simulink model "amicas_simulator_v1"  (R2024b)
settings: Solver=ode3  StartTime=0.0  StopTime=Tsim  FixedStep=ST  RelTol=1e-3
values from neighbouring files (symbols this model uses):
  alpha_GN = 7.76    [amicas_anesthesia_model.m]
  alpha_RG = 0.33    [amicas_anesthesia_model.m]
  alpha_RGN = 1.61    [amicas_anesthesia_model.m]
  Anest_loop = 1    [amicas_main_program.m]
  Ap = sys11.A    [amicas_estimation_adaptation.m]
  Ar = sys12.A    [amicas_estimation_adaptation.m]
  beta_M = 10.74    [amicas_anesthesia_model.m]
  beta_MN = 3.36    [amicas_anesthesia_model.m]
  Bp = sys11.B    [amicas_estimation_adaptation.m]
  Br = sys12.B    [amicas_estimation_adaptation.m]
  C50N = 3.2425    [amicas_anesthesia_model.m]
  C50P_GN = 1273.3    [amicas_anesthesia_model.m]
  C50P_M = 7.53    [amicas_anesthesia_model.m]
  C50P_MN = 1188.7    [amicas_anesthesia_model.m]
  C50P_RG = 8.26    [amicas_anesthesia_model.m]
  C50P_RGN = 67.77    [amicas_anesthesia_model.m]
  C50Pco = 8    [amicas_hemodyn_model.m]
  C50Pmap = 6    [amicas_hemodyn_model.m]
  C50R_GN = 8.30    (= 8.3)    [amicas_anesthesia_model.m]
  C50R_M = 160.25    [amicas_anesthesia_model.m]
  C50R_MN = 14.64    [amicas_anesthesia_model.m]
  C50Rco = 12    [amicas_hemodyn_model.m]
  C50Rmap = 17    [amicas_hemodyn_model.m]
  Cobasis = 5    [amicas_hemodyn_model.m]
  Cp = sys11.C    [amicas_estimation_adaptation.m]
  Cr = sys12.C    [amicas_estimation_adaptation.m]
  Dist_type = 1    [amicas_main_program.m]
  E0_G = 93.97    [amicas_anesthesia_model.m]
  E0_GN = 33.34    [amicas_anesthesia_model.m]
  E0_M = 93.97    [amicas_anesthesia_model.m]
  E0_MN = 34.48    [amicas_anesthesia_model.m]
  E0_RG = 93.97    [amicas_anesthesia_model.m]
  E0_RGN = 33.69    [amicas_anesthesia_model.m]
  Emax_G = E0_G    (= 93.97)    [amicas_anesthesia_model.m]
  Emax_GN = E0_GN    (= 33.34)    [amicas_anesthesia_model.m]
  Emax_M = E0_M    (= 93.97)    [amicas_anesthesia_model.m]
  Emax_MN = E0_MN    (= 34.48)    [amicas_anesthesia_model.m]
  Emax_RG = E0_RG    (= 93.97)    [amicas_anesthesia_model.m]
  Emax_RGN = E0_RGN    (= 33.69)    [amicas_anesthesia_model.m]
  EmaxPco = 5    [amicas_hemodyn_model.m]
  EmaxPmap = 5    [amicas_hemodyn_model.m]
  EmaxRco = 5    [amicas_hemodyn_model.m]
  EmaxRmap = 15    [amicas_hemodyn_model.m]
  gainPco = 10    [amicas_hemodyn_model.m]
  gainPmap = 15    [amicas_hemodyn_model.m]
  gainRco = 10    [amicas_hemodyn_model.m]
  gainRmap = 10    [amicas_hemodyn_model.m]
  gamma_GN = 7.14    [amicas_anesthesia_model.m]
  gamma_M = 4.13    [amicas_anesthesia_model.m]
  gamma_MN = 6.56    [amicas_anesthesia_model.m]
  gamma_RG = 3.59    [amicas_anesthesia_model.m]
  gamma_RGN = 5.34    [amicas_anesthesia_model.m]
  gammaN = 2.6677    [amicas_anesthesia_model.m]
  gammaPco = 4.5    [amicas_hemodyn_model.m]
  gammaPmap = 4.5    [amicas_hemodyn_model.m]
  gammaRco = 4.5    [amicas_hemodyn_model.m]
  gammaRmap = 4.5    [amicas_hemodyn_model.m]
  k0Pco = 0.81    [amicas_hemodyn_model.m]
  k0Pmap = 0.81    [amicas_hemodyn_model.m]
  k0Rco = 0.51    [amicas_hemodyn_model.m]
  k0Rmap = 0.31    [amicas_hemodyn_model.m]
  k1Pco = 0.81/60    (= 0.0135)    [amicas_hemodyn_model.m]
  k1Pmap = 0.61/60    (= 0.0101666666667)    [amicas_hemodyn_model.m]
  k1Rco = 0.51/60    (= 0.0085)    [amicas_hemodyn_model.m]
  k1Rmap = 0.31/60    (= 0.00516666666667)    [amicas_hemodyn_model.m]
  MAPbasis = 80    [amicas_hemodyn_model.m]
  patient = Patients(index)    [amicas_main_program.m]
  RSM_type = 3    [amicas_main_program.m]
  Ts = 1/60    (= 0.0166666666667)    [amicas_main_program.m]
  Tsc = 5/60    (= 0.0833333333333)    [amicas_estimation_adaptation.m]
libraries: cstblocks x12
settings Model: Creator=Merigo  LastModifiedBy=erhan
settings SolverCC: AlgebraicLoopSolver=TrustRegion
settings DataIOCC: LimitDataPoints=on  SaveFormat=Array  SignalLoggingSaveFormat=ModelDataLogs  ReturnWorkspaceOutputs=off
settings OptimizationCC: BlockReduction=off  BooleanDataType=off  ReuseModelBlockBuffer=off  ExpressionDepthLimit=2147483647  LifeSpan=inf
settings DebuggingCC: SaveWithParameterizedLinksMsg=none  UnderspecifiedInitializationDetection=Classic  MergeDetectMultiDrivingBlocksExec=none  SignalResolutionControl=TryResolveAllWithWarning  MultiTaskDSMMsg=warning  MultiTaskCondExecSysMsg=none  UnconnectedInputMsg=warning  UnconnectedOutputMsg=warning  UnconnectedLineMsg=warning  StateNameClashWarn=warning  SFUnexpectedBacktrackingDiag=warning  SFNoUnconditionalDefaultTransitionDiag=warning  SFExecutionAtInitializationDiag=none  ArithmeticOperatorsInVariantConditions=warning
settings HardwareCC: ProdBitPerPointer=32  ProdBitPerSizeT=32  ProdBitPerPtrDiffT=32  ProdLargestAtomicFloat=None  ProdIntDivRoundTo=Undefined  ProdEndianess=Unspecified  ProdWordSize=32  ProdHWDeviceType=32-bit Generic  TargetUnknown=on
settings ModelReferenceCC: EnableRefExpFcnMdlSchedulingChecks=on  PropagateSignalLabelsOutOfModel=off
settings SFSimCC: SimUseLocalCustomCode=off  CustomCodeUndefinedFunction=UseInterfaceOnly
settings RTWCC: RTWUseLocalCustomCode=off  GPUComputeCapability=3.5  DLArmComputeVersion=19.05
settings CodeAppCC: StateflowObjectComments=on
settings GRTTargetCC: TargetLangStandard=C89/C90 (ANSI)
settings ConfigComp: CovMetricSettings=dw  CovSaveCumulativeToWorkspaceVar=on  CovSaveSingleToWorkspaceVar=on  CovExternalEMLEnable=off

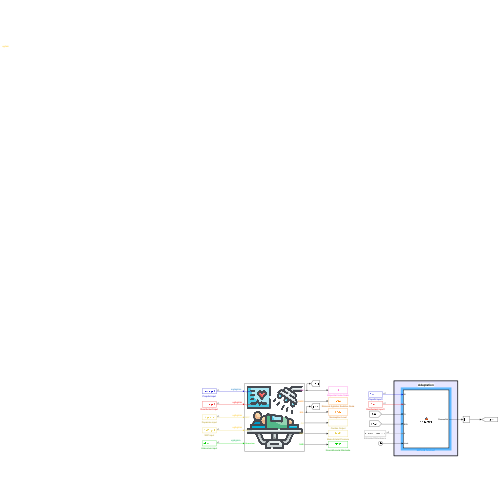
[thumbnail: Simulink's stored preview of the top-level diagram]
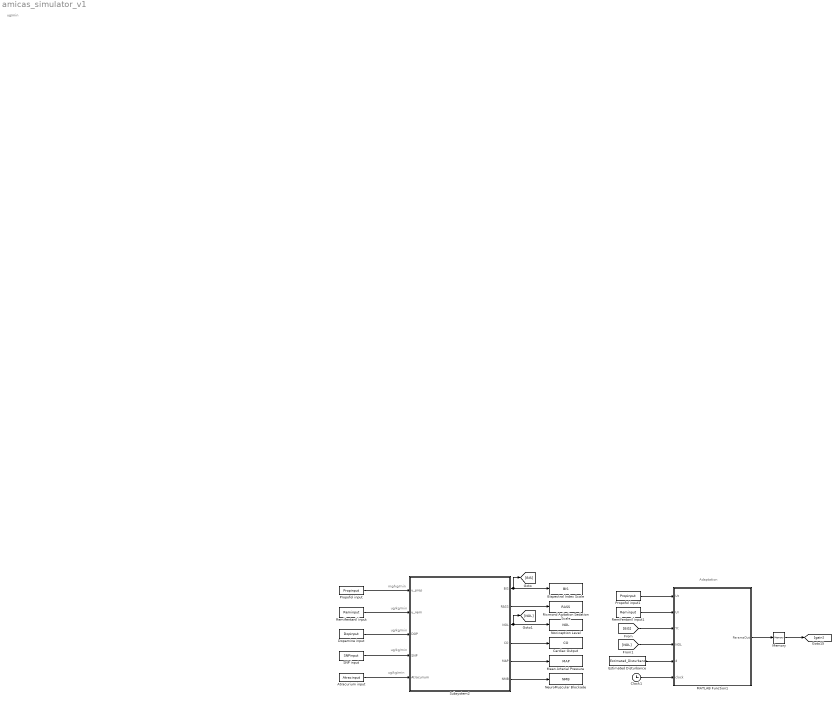
== system amicas_simulator_v1 ==
  note: ug/kg/min
  note: mg/kg/min
  note: ug/min
  note: ug/kg/min
  note: ug/kg/min
  note: ug/kg/min
  note: Adaptation
  Atracurium input : FromWorkspace  VariableName=Atracinput  Interpolate=off  OutputAfterFinalValue=Setting to zero
  Bispectral Index Scale : ToWorkspace  VariableName=BIS  SaveFormat=Timeseries  SampleTime=-1
  Cardiac Output : ToWorkspace  VariableName=CO  SaveFormat=Timeseries  SampleTime=-1
  Clock1 : Clock
  Dopamine input : FromWorkspace  VariableName=Dopinput  Interpolate=off  OutputAfterFinalValue=Setting to zero
  Estimated Disturbance : FromWorkspace  VariableName=Estimated_Disturbance  Interpolate=off  OutputAfterFinalValue=Setting to zero
  MATLAB Function1 : MATLAB Function  TreatAsAtomicUnit=on  SystemSampleTime=Tsc
  Mean Arterial Pressure : ToWorkspace  VariableName=MAP  SaveFormat=Timeseries  SampleTime=-1
  Memory : Memory
  NeuroMuscular Blockade : ToWorkspace  VariableName=NMB  SaveFormat=Timeseries  SampleTime=-1
  Nociception Level : ToWorkspace  VariableName=NOL  SaveFormat=Timeseries  SampleTime=-1
  Propofol input : FromWorkspace  VariableName=Propinput  Interpolate=off  OutputAfterFinalValue=Setting to zero
  Propofol input1 : FromWorkspace  VariableName=Propinput  Interpolate=off  OutputAfterFinalValue=Setting to zero
  Remifentanil input : FromWorkspace  VariableName=Reminput  Interpolate=off  OutputAfterFinalValue=Setting to zero
  Remifentanil input1 : FromWorkspace  VariableName=Reminput  Interpolate=off  OutputAfterFinalValue=Setting to zero
  Ricmond Agitation Sedation Scale : ToWorkspace  VariableName=RASS  SaveFormat=Timeseries  SampleTime=-1
  SNP input : FromWorkspace  VariableName=SNPinput  Interpolate=off  OutputAfterFinalValue=Setting to zero
  Subsystem2 : Subsystem
      mask Display: image('$imagefile');
  wires:
  Propofol input/1 -> Subsystem2/1(u_prop)
  Subsystem2/2(RASS) -> Ricmond Agitation Sedation Scale/1
  Subsystem2/4(CO) -> Cardiac Output/1
  Subsystem2/5(MAP) -> Mean Arterial Pressure/1
  Subsystem2/6(NMB) -> NeuroMuscular Blockade/1
  Atracurium input/1 -> Subsystem2/5(Atracurium)
  Subsystem2/1(BIS) -> Bispectral Index Scale/1, [BIS]
  Remifentanil input/1 -> Subsystem2/2(u_remi)
  Dopamine input/1 -> Subsystem2/3(DOP)
  SNP input/1 -> Subsystem2/4(SNP)
  Subsystem2/3(NOL) -> Nociception Level/1, [NOL]
  [NOL] -> MATLAB Function1/4(NOL)
  [BIS] -> MATLAB Function1/3(Yt)
  Propofol input1/1 -> MATLAB Function1/1(Ut)
  Memory/1 -> [gain]
  MATLAB Function1/1(ParamsOut) -> Memory/1
  Clock1/1 -> MATLAB Function1/6(clock)
  Estimated Disturbance/1 -> MATLAB Function1/5(d)
  Remifentanil input1/1 -> MATLAB Function1/2(Ur)

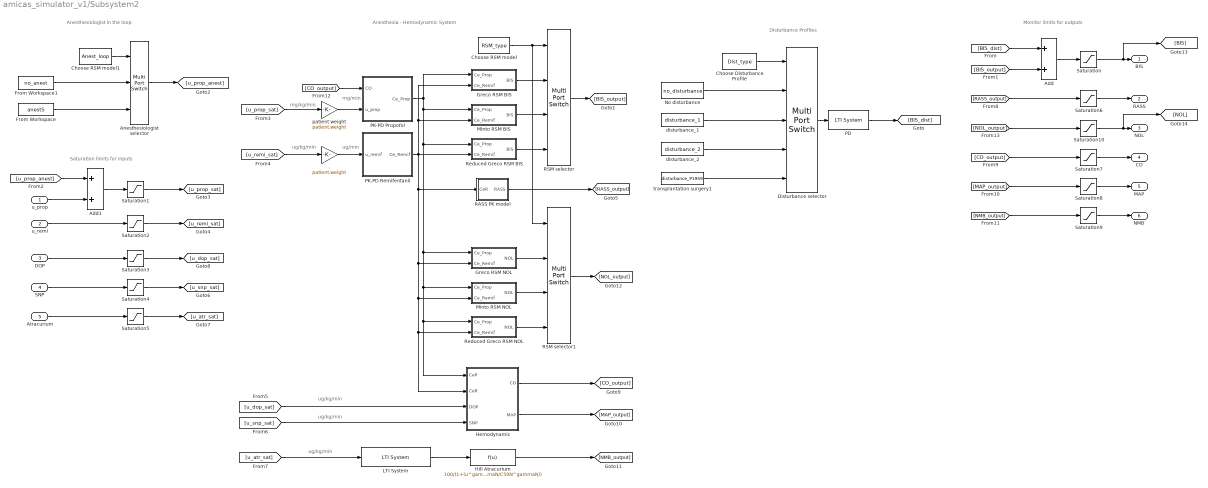
== system amicas_simulator_v1/Subsystem2 ==
  note: Disturbance Profiles
  note: Anesthesia - Hemodynamic System
  note: ug/kg/min
  note: ug/kg/min
  note: ug/kg/min
  note: ug/kg/min
  note: mg/kg/min
  note: Anesthesiologist in the loop
  note: ug/min
  note: mg/min
  note: Saturation limits for inputs
  note: Monitor limits for outputs
  u_prop : Inport
  u_remi : Inport  Port=2
  DOP : Inport  Port=3
  SNP : Inport  Port=4
  Atracurium : Inport  Port=5
  . : Gain  Gain=patient.weight
  Add : Sum
  Add1 : Sum
  Anesthesiologist selector : MultiPortSwitch  DataPortOrder=Specify indices  Inputs=2  DataPortIndices={1,2}  SaturateOnIntegerOverflow=off  InputSameDT=off
  Choose Disturbance Profile : Constant  Value=Dist_type
  Choose RSM model : Constant  Value=RSM_type
  Choose RSM model1 : Constant  Value=Anest_loop
  Disturbance selector : MultiPortSwitch  DataPortOrder=Specify indices  Inputs=10  DataPortIndices={1,2,3,4}  SaturateOnIntegerOverflow=off  InputSameDT=off
  From Workspace : FromWorkspace  VariableName=anestS
  From Workspace1 : FromWorkspace  VariableName=no_anest
  Greco RSM BIS : Subsystem
  Greco RSM NOL : Subsystem
  Hemodynamic : Subsystem
  Hill Atracurium : Fcn  Expr=100/(1+(u^gammaN/C50N^gammaN))
  LTI System : cstblocks/LTI System  sys=sysNMB  IC=[]  PadeOrder=0
  Minto RSM BIS : Subsystem
  Minto RSM NOL : Subsystem
  No disturbance : FromWorkspace  VariableName=no_disturbance  Interpolate=off  OutputAfterFinalValue=Setting to zero
  PD : cstblocks/LTI System  sys=CPmodelP  IC=[]  PadeOrder=0
  PK-PD Propofol : Subsystem
  PK-PD Remifentanil : Subsystem
  RASS PK model : Subsystem
  RSM selector : MultiPortSwitch  DataPortOrder=Specify indices  SaturateOnIntegerOverflow=off  InputSameDT=off
  RSM selector1 : MultiPortSwitch  DataPortOrder=Specify indices  SaturateOnIntegerOverflow=off  InputSameDT=off
  Reduced Greco RSM BIS : Subsystem
  Reduced Greco RSM NOL : Subsystem
  Saturation : Saturate  UpperLimit=100  LowerLimit=0
  Saturation1 : Saturate  UpperLimit=2.5  LowerLimit=0
  Saturation10 : Saturate  UpperLimit=100  LowerLimit=0
  Saturation2 : Saturate  UpperLimit=4  LowerLimit=0
  Saturation3 : Saturate  UpperLimit=20  LowerLimit=0
  Saturation4 : Saturate  UpperLimit=10  LowerLimit=0
  Saturation5 : Saturate  UpperLimit=29.5  LowerLimit=0
  Saturation6 : Saturate  UpperLimit=4  LowerLimit=-5
  Saturation7 : Saturate  UpperLimit=40  LowerLimit=0
  Saturation8 : Saturate  UpperLimit=150  LowerLimit=0
  Saturation9 : Saturate  UpperLimit=100  LowerLimit=0
  disturbance_1 : FromWorkspace  VariableName=disturbance_1  Interpolate=off  OutputAfterFinalValue=Setting to zero
  disturbance_2 : FromWorkspace  VariableName=disturbance_2  Interpolate=off  OutputAfterFinalValue=Setting to zero
  patient weight : Gain  Gain=patient.weight
  transplantation surgery1 : FromWorkspace  VariableName=disturbance_P1959  Interpolate=off  OutputAfterFinalValue=Setting to zero
  BIS : Outport
  RASS : Outport  Port=2
  NOL : Outport  Port=3
  CO : Outport  Port=4
  MAP : Outport  Port=5
  NMB : Outport  Port=6
  wires:
  PK-PD Remifentanil/1(Ce_Remif) -> Minto RSM BIS/2(Ce_Remif), Greco RSM BIS/2(Ce_Remif), Greco RSM NOL/2(Ce_Remif), Minto RSM NOL/2(Ce_Remif), Reduced Greco RSM NOL/2(Ce_Remif), Hemodynamic/2(CeR), RASS PK model/1(CeR), Reduced Greco RSM BIS/2(Ce_Remif)
  PK-PD Propofol/1(Ce_Prop) -> Greco RSM NOL/1(Ce_Prop), Minto RSM NOL/1(Ce_Prop), Reduced Greco RSM NOL/1(Ce_Prop), Hemodynamic/1(CeP), Reduced Greco RSM BIS/1(Ce_Prop), Minto RSM BIS/1(Ce_Prop), Greco RSM BIS/1(Ce_Prop)
  RASS PK model/1(RASS) -> [RASS_output]
  Hill Atracurium/1 -> [NMB_output]
  [u_atr_sat] -> LTI System/1
  LTI System/1 -> Hill Atracurium/1
  [u_dop_sat] -> Hemodynamic/3(DOP)
  [u_snp_sat] -> Hemodynamic/4(SNP)
  Hemodynamic/1(CO) -> [CO_output]
  Hemodynamic/2(MAP) -> [MAP_output]
  From Workspace/1 -> Anesthesiologist selector/3
  [u_remi_sat] -> ./1
  Reduced Greco RSM BIS/1(BIS) -> RSM selector/4
  Greco RSM BIS/1(BIS) -> RSM selector/2
  Minto RSM BIS/1(BIS) -> RSM selector/3
  RSM selector/1 -> [BIS_output]
  Choose RSM model/1 -> RSM selector1/1, RSM selector/1
  Add/1 -> Saturation/1
  Disturbance selector/1 -> PD/1
  No disturbance/1 -> Disturbance selector/2
  [BIS_dist] -> Add/1
  disturbance_1/1 -> Disturbance selector/3
  Choose Disturbance Profile/1 -> Disturbance selector/1
  PD/1 -> [BIS_dist]
  [BIS_output] -> Add/2
  Choose RSM model1/1 -> Anesthesiologist selector/1
  Anesthesiologist selector/1 -> [u_prop_anest]
  From Workspace1/1 -> Anesthesiologist selector/2
  disturbance_2/1 -> Disturbance selector/4
  [u_prop_sat] -> patient weight/1
  ./1 -> PK-PD Remifentanil/1(u_remif)
  patient weight/1 -> PK-PD Propofol/2(u_prop)
  Saturation/1 -> [BIS], BIS/1
  u_prop/1 -> Add1/2
  Saturation1/1 -> [u_prop_sat]
  Add1/1 -> Saturation1/1
  [u_prop_anest] -> Add1/1
  u_remi/1 -> Saturation2/1
  Saturation2/1 -> [u_remi_sat]
  Saturation3/1 -> [u_dop_sat]
  DOP/1 -> Saturation3/1
  SNP/1 -> Saturation4/1
  Saturation4/1 -> [u_snp_sat]
  Atracurium/1 -> Saturation5/1
  Saturation5/1 -> [u_atr_sat]
  [RASS_output] -> Saturation6/1
  Saturation6/1 -> RASS/1
  Saturation7/1 -> CO/1
  [CO_output] -> Saturation7/1
  Saturation8/1 -> MAP/1
  [MAP_output] -> Saturation8/1
  Saturation9/1 -> NMB/1
  [NMB_output] -> Saturation9/1
  [CO_output] -> PK-PD Propofol/1(CO)
  Greco RSM NOL/1(NOL) -> RSM selector1/2
  Minto RSM NOL/1(NOL) -> RSM selector1/3
  Reduced Greco RSM NOL/1(NOL) -> RSM selector1/4
  RSM selector1/1 -> [NOL_output]
  [NOL_output] -> Saturation10/1
  Saturation10/1 -> [NOL], NOL/1
  transplantation surgery1/1 -> Disturbance selector/5

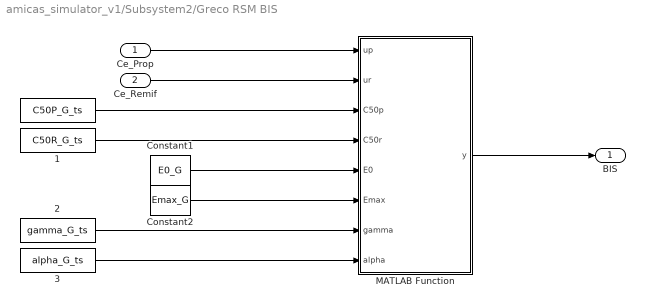
== system amicas_simulator_v1/Subsystem2/Greco RSM BIS ==
  Ce_Prop : Inport
  Ce_Remif : Inport  Port=2
  " " : FromWorkspace  VariableName=C50P_G_ts  Interpolate=off  OutputAfterFinalValue=Setting to zero
  " 1" : FromWorkspace  VariableName=C50R_G_ts  Interpolate=off  OutputAfterFinalValue=Setting to zero
  " 2" : FromWorkspace  VariableName=gamma_G_ts  Interpolate=off  OutputAfterFinalValue=Setting to zero
  " 3" : FromWorkspace  VariableName=alpha_G_ts  Interpolate=off  OutputAfterFinalValue=Setting to zero
  Constant1 : Constant  Value=E0_G
  Constant2 : Constant  Value=Emax_G
  MATLAB Function : MATLAB Function  TreatAsAtomicUnit=on
  BIS : Outport
  wires:
  Ce_Remif/1 -> MATLAB Function/2(ur)
  " "/1 -> MATLAB Function/3(C50p)
  Ce_Prop/1 -> MATLAB Function/1(up)
  " 2"/1 -> MATLAB Function/7(gamma)
  Constant1/1 -> MATLAB Function/5(E0)
  " 1"/1 -> MATLAB Function/4(C50r)
  Constant2/1 -> MATLAB Function/6(Emax)
  " 3"/1 -> MATLAB Function/8(alpha)
  MATLAB Function/1(y) -> BIS/1

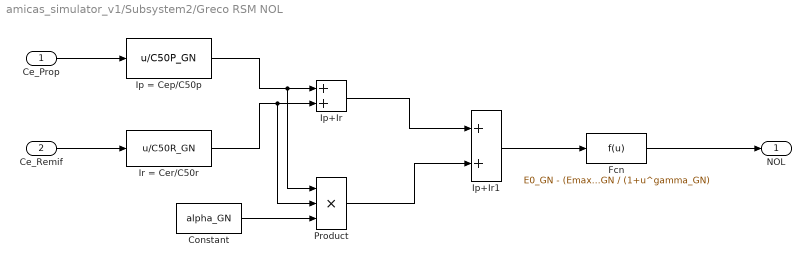
== system amicas_simulator_v1/Subsystem2/Greco RSM NOL ==
  Ce_Prop : Inport
  Ce_Remif : Inport  Port=2
  Constant : Constant  Value=alpha_GN
  Fcn : Fcn  Expr=E0_GN - (Emax_GN) * u^gamma_GN / (1+u^gamma_GN)
  Ip = Cep/C50p : Fcn  Expr=u/C50P_GN
  Ip+Ir : Sum
  Ip+Ir1 : Sum
  Ir = Cer/C50r : Fcn  Expr=u/C50R_GN
  Product : Product  Inputs=3
  NOL : Outport
  wires:
  Fcn/1 -> NOL/1
  Ip+Ir1/1 -> Fcn/1
  Ir = Cer/C50r/1 -> Product/2, Ip+Ir/2
  Ip = Cep/C50p/1 -> Product/1, Ip+Ir/1
  Ce_Remif/1 -> Ir = Cer/C50r/1
  Ce_Prop/1 -> Ip = Cep/C50p/1
  Ip+Ir/1 -> Ip+Ir1/1
  Constant/1 -> Product/3
  Product/1 -> Ip+Ir1/2

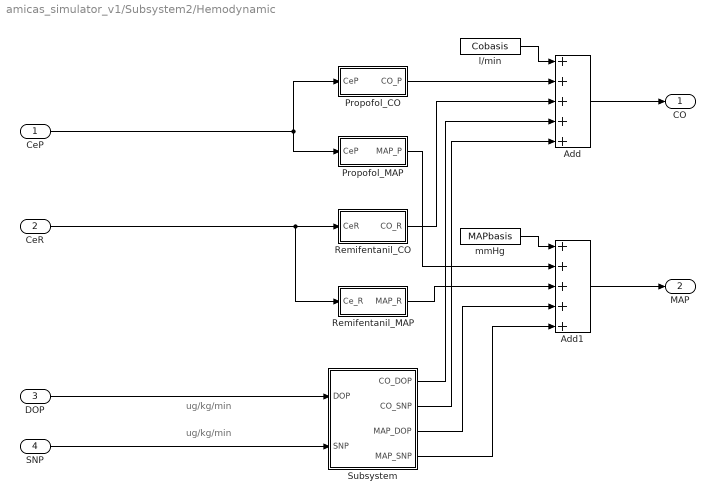
== system amicas_simulator_v1/Subsystem2/Hemodynamic ==
  note: ug/kg/min
  note: ug/kg/min
  CeP : Inport
  CeR : Inport  Port=2
  DOP : Inport  Port=3
  SNP : Inport  Port=4
  Add : Sum  Inputs=+++++
  Add1 : Sum  Inputs=+++++
  Propofol_CO : Subsystem
  Propofol_MAP : Subsystem
  Remifentanil_CO : Subsystem
  Remifentanil_MAP : Subsystem
  Subsystem : Subsystem
  l/min : Constant  Value=Cobasis  SampleTime=Ts
  mmHg : Constant  Value=MAPbasis  SampleTime=Ts
  CO : Outport
  MAP : Outport  Port=2
  wires:
  DOP/1 -> Subsystem/1(DOP)
  SNP/1 -> Subsystem/2(SNP)
  Subsystem/1(CO_DOP) -> Add/4
  Propofol_CO/1(CO_P) -> Add/2
  Subsystem/3(MAP_DOP) -> Add1/4
  CeP/1 -> Propofol_CO/1(CeP), Propofol_MAP/1(CeP)
  Subsystem/2(CO_SNP) -> Add/5
  CeR/1 -> Remifentanil_MAP/1(Ce_R), Remifentanil_CO/1(CeR)
  Propofol_MAP/1(MAP_P) -> Add1/2
  Remifentanil_CO/1(CO_R) -> Add/3
  Add/1 -> CO/1
  Add1/1 -> MAP/1
  mmHg/1 -> Add1/1
  Subsystem/4(MAP_SNP) -> Add1/5
  l/min/1 -> Add/1
  Remifentanil_MAP/1(MAP_R) -> Add1/3

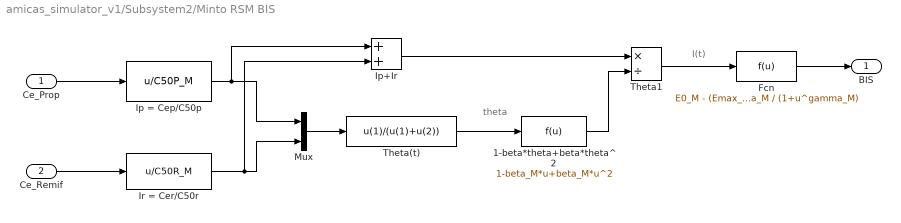
== system amicas_simulator_v1/Subsystem2/Minto RSM BIS ==
  note: I(t)
  note: theta
  Ce_Prop : Inport
  Ce_Remif : Inport  Port=2
  1-beta*theta+beta*theta^2 : Fcn  Expr=1-beta_M*u+beta_M*u^2
  Fcn : Fcn  Expr=E0_M - (Emax_M)*u^gamma_M / (1+u^gamma_M)
  Ip = Cep/C50p : Fcn  Expr=u/C50P_M
  Ip+Ir : Sum
  Ir = Cer/C50r : Fcn  Expr=u/C50R_M
  Mux : Mux  Inputs=2
  Theta(t) : Fcn  Expr=u(1)/(u(1)+u(2))
  Theta1 : Product  Inputs=*/
  BIS : Outport
  wires:
  Ce_Prop/1 -> Ip = Cep/C50p/1
  Ce_Remif/1 -> Ir = Cer/C50r/1
  Ip = Cep/C50p/1 -> Mux/1, Ip+Ir/1
  Ir = Cer/C50r/1 -> Mux/2, Ip+Ir/2
  Mux/1 -> Theta(t)/1
  Ip+Ir/1 -> Theta1/1
  Theta(t)/1 -> 1-beta*theta+beta*theta^2/1
  1-beta*theta+beta*theta^2/1 -> Theta1/2
  Theta1/1 -> Fcn/1
  Fcn/1 -> BIS/1

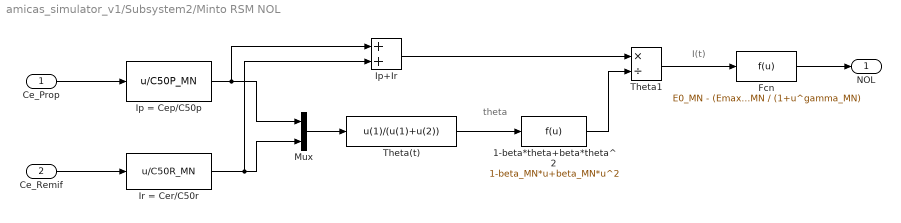
== system amicas_simulator_v1/Subsystem2/Minto RSM NOL ==
  note: I(t)
  note: theta
  Ce_Prop : Inport
  Ce_Remif : Inport  Port=2
  1-beta*theta+beta*theta^2 : Fcn  Expr=1-beta_MN*u+beta_MN*u^2
  Fcn : Fcn  Expr=E0_MN - (Emax_MN)*u^gamma_MN / (1+u^gamma_MN)
  Ip = Cep/C50p : Fcn  Expr=u/C50P_MN
  Ip+Ir : Sum
  Ir = Cer/C50r : Fcn  Expr=u/C50R_MN
  Mux : Mux  Inputs=2
  Theta(t) : Fcn  Expr=u(1)/(u(1)+u(2))
  Theta1 : Product  Inputs=*/
  NOL : Outport
  wires:
  Ce_Prop/1 -> Ip = Cep/C50p/1
  Ce_Remif/1 -> Ir = Cer/C50r/1
  Ip = Cep/C50p/1 -> Mux/1, Ip+Ir/1
  Ir = Cer/C50r/1 -> Mux/2, Ip+Ir/2
  Mux/1 -> Theta(t)/1
  Ip+Ir/1 -> Theta1/1
  Theta(t)/1 -> 1-beta*theta+beta*theta^2/1
  1-beta*theta+beta*theta^2/1 -> Theta1/2
  Theta1/1 -> Fcn/1
  Fcn/1 -> NOL/1

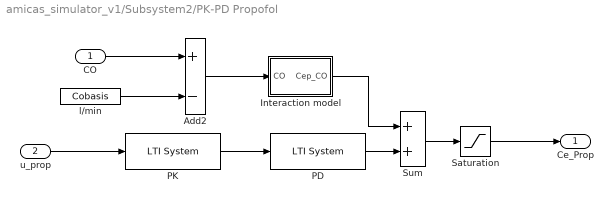
== system amicas_simulator_v1/Subsystem2/PK-PD Propofol ==
  CO : Inport
  u_prop : Inport  Port=2
  Add2 : Sum  Inputs=+-
  Interaction model : Subsystem
  PD : cstblocks/LTI System  sys=CPmodelP  IC=[]  PadeOrder=0
  PK : cstblocks/LTI System  sys=PKmodelP  IC=[]  PadeOrder=0
  Saturation : Saturate  UpperLimit=Inf  LowerLimit=0.001  ZeroCross=off
  Sum : Sum
  l/min : Constant  Value=Cobasis  SampleTime=Ts
  Ce_Prop : Outport
  wires:
  u_prop/1 -> PK/1
  PD/1 -> Sum/2
  PK/1 -> PD/1
  Saturation/1 -> Ce_Prop/1
  l/min/1 -> Add2/2
  Add2/1 -> Interaction model/1(CO)
  Sum/1 -> Saturation/1
  CO/1 -> Add2/1
  Interaction model/1(Cep_CO) -> Sum/1

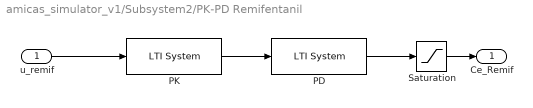
== system amicas_simulator_v1/Subsystem2/PK-PD Remifentanil ==
  u_remif : Inport
  PD : cstblocks/LTI System  sys=CPmodelR  IC=[]  PadeOrder=0
  PK : cstblocks/LTI System  sys=PKmodelR  IC=[]  PadeOrder=0
  Saturation : Saturate  UpperLimit=Inf  LowerLimit=0.001  ZeroCross=off
  Ce_Remif : Outport
  wires:
  PK/1 -> PD/1
  u_remif/1 -> PK/1
  PD/1 -> Saturation/1
  Saturation/1 -> Ce_Remif/1

== system amicas_simulator_v1/Subsystem2/RASS PK model ==
  CeR : Inport
  LTI System : cstblocks/LTI System  sys=sysRASS1  IC=[]  PadeOrder=0
  LTI System1 : cstblocks/LTI System  sys=sysRASS2  IC=[]  PadeOrder=0
  RASS : Outport
  wires:
  CeR/1 -> LTI System/1
  LTI System/1 -> LTI System1/1
  LTI System1/1 -> RASS/1

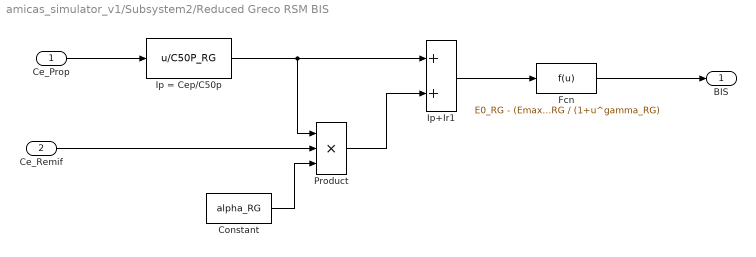
== system amicas_simulator_v1/Subsystem2/Reduced Greco RSM BIS ==
  Ce_Prop : Inport
  Ce_Remif : Inport  Port=2
  Constant : Constant  Value=alpha_RG
  Fcn : Fcn  Expr=E0_RG - (Emax_RG ) * u^gamma_RG / (1+u^gamma_RG)
  Ip = Cep/C50p : Fcn  Expr=u/C50P_RG
  Ip+Ir1 : Sum
  Product : Product  Inputs=3
  BIS : Outport
  wires:
  Fcn/1 -> BIS/1
  Ip+Ir1/1 -> Fcn/1
  Ce_Remif/1 -> Product/2
  Ce_Prop/1 -> Ip = Cep/C50p/1
  Ip = Cep/C50p/1 -> Product/1, Ip+Ir1/1
  Constant/1 -> Product/3
  Product/1 -> Ip+Ir1/2

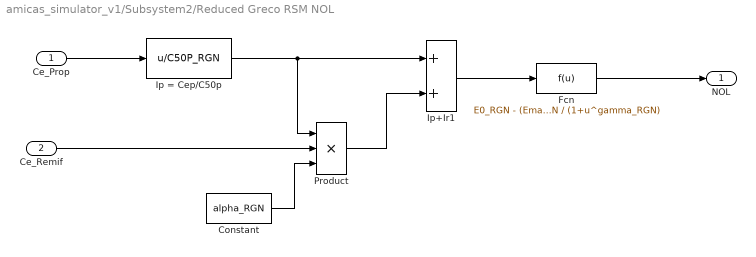
== system amicas_simulator_v1/Subsystem2/Reduced Greco RSM NOL ==
  Ce_Prop : Inport
  Ce_Remif : Inport  Port=2
  Constant : Constant  Value=alpha_RGN
  Fcn : Fcn  Expr=E0_RGN - (Emax_RGN) * u^gamma_RGN / (1+u^gamma_RGN)
  Ip = Cep/C50p : Fcn  Expr=u/C50P_RGN
  Ip+Ir1 : Sum
  Product : Product  Inputs=3
  NOL : Outport
  wires:
  Fcn/1 -> NOL/1
  Ip+Ir1/1 -> Fcn/1
  Ce_Remif/1 -> Product/2
  Ce_Prop/1 -> Ip = Cep/C50p/1
  Ip = Cep/C50p/1 -> Product/1, Ip+Ir1/1
  Constant/1 -> Product/3
  Product/1 -> Ip+Ir1/2

== system amicas_simulator_v1/Subsystem2/Hemodynamic/Propofol_CO ==
  CeP : Inport
  Hill prop to CO : Fcn  Expr=-(EmaxPco*(u^gammaPco/(u^gammaPco+C50Pco^gammaPco)))
  MAP PK model : Subsystem
  CO_P : Outport  VectorParamsAs1DForOutWhenUnconnected=off
  wires:
  MAP PK model/1(CO) -> Hill prop to CO/1
  CeP/1 -> MAP PK model/1(CeP)
  Hill prop to CO/1 -> CO_P/1

== system amicas_simulator_v1/Subsystem2/Hemodynamic/Propofol_MAP ==
  CeP : Inport
  Hill Prop to MAP1 : Fcn  Expr=-(EmaxPmap*(u^gammaPmap/(u^gammaPmap+C50Pmap^gammaPmap)))
  MAP PK model1 : Subsystem
  MAP_P : Outport  VectorParamsAs1DForOutWhenUnconnected=off
  wires:
  MAP PK model1/1(MAP) -> Hill Prop to MAP1/1
  CeP/1 -> MAP PK model1/1(CeP)
  Hill Prop to MAP1/1 -> MAP_P/1

== system amicas_simulator_v1/Subsystem2/Hemodynamic/Remifentanil_CO ==
  CeR : Inport
  Hill Remifentanil to CO : Fcn  Expr=EmaxRco*(u^gammaRco/(u^gammaRco+C50Rco^gammaRco))
  MAP PK model2 : Subsystem
  CO_R : Outport  VectorParamsAs1DForOutWhenUnconnected=off
  wires:
  CeR/1 -> MAP PK model2/1(CeR)
  MAP PK model2/1(CO) -> Hill Remifentanil to CO/1
  Hill Remifentanil to CO/1 -> CO_R/1

== system amicas_simulator_v1/Subsystem2/Hemodynamic/Remifentanil_MAP ==
  Ce_R : Inport
  Hill Remi MAP : Fcn  Expr=-(EmaxRmap*(u^gammaRmap/(u^gammaRmap+C50Rmap^gammaRmap)))
  MAP PK model3 : Subsystem
  MAP_R : Outport  VectorParamsAs1DForOutWhenUnconnected=off
  wires:
  Ce_R/1 -> MAP PK model3/1(CeR)
  MAP PK model3/1(MAP) -> Hill Remi MAP/1
  Hill Remi MAP/1 -> MAP_R/1

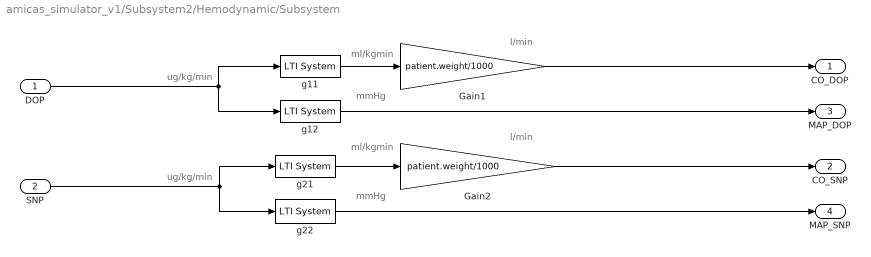
== system amicas_simulator_v1/Subsystem2/Hemodynamic/Subsystem ==
  note: ml/kgmin
  note: l/min
  note: ug/kg/min
  note: mmHg
  note: mmHg
  note: ug/kg/min
  note: ml/kgmin
  note: l/min
  DOP : Inport
  SNP : Inport  Port=2
  Gain1 : Gain  Gain=patient.weight/1000
  Gain2 : Gain  Gain=patient.weight/1000
  g11 : cstblocks/LTI System  sys=g11  IC=[]  PadeOrder=0
  g12 : cstblocks/LTI System  sys=g12  IC=[]  PadeOrder=0
  g21 : cstblocks/LTI System  sys=g21  IC=[]  PadeOrder=0
  g22 : cstblocks/LTI System  sys=g22  IC=[]  PadeOrder=0
  CO_DOP : Outport
  CO_SNP : Outport  Port=2
  MAP_DOP : Outport  Port=3
  MAP_SNP : Outport  Port=4
  wires:
  Gain1/1 -> CO_DOP/1
  SNP/1 -> g22/1, g21/1
  g12/1 -> MAP_DOP/1
  g22/1 -> MAP_SNP/1
  g21/1 -> Gain2/1
  DOP/1 -> g12/1, g11/1
  g11/1 -> Gain1/1
  Gain2/1 -> CO_SNP/1

== system amicas_simulator_v1/Subsystem2/PK-PD Propofol/Interaction model ==
  CO : Inport
  Transfer Fcn : TransferFcn  Numerator=[-0.35]  Denominator=[300 1]
  Cep_CO : Outport
  wires:
  CO/1 -> Transfer Fcn/1
  Transfer Fcn/1 -> Cep_CO/1

== system amicas_simulator_v1/Subsystem2/Hemodynamic/Propofol_CO/MAP PK model ==
  CeP : Inport
  Transfer Fcn : TransferFcn  Numerator=[0.7]  Denominator=[k1Pco*gainPco k0Pco]
  CO : Outport
  wires:
  Transfer Fcn/1 -> CO/1
  CeP/1 -> Transfer Fcn/1

== system amicas_simulator_v1/Subsystem2/Hemodynamic/Propofol_MAP/MAP PK model1 ==
  CeP : Inport
  Transfer Fcn : TransferFcn  Denominator=[k1Pmap*gainPmap k0Pmap]
  MAP : Outport
  wires:
  Transfer Fcn/1 -> MAP/1
  CeP/1 -> Transfer Fcn/1

== system amicas_simulator_v1/Subsystem2/Hemodynamic/Remifentanil_CO/MAP PK model2 ==
  CeR : Inport
  Transfer Fcn : TransferFcn  Denominator=[k1Rco*gainRco k0Rco]
  CO : Outport
  wires:
  Transfer Fcn/1 -> CO/1
  CeR/1 -> Transfer Fcn/1

== system amicas_simulator_v1/Subsystem2/Hemodynamic/Remifentanil_MAP/MAP PK model3 ==
  CeR : Inport
  Transfer Fcn : TransferFcn  Denominator=[k1Rmap*gainRmap k0Rmap]
  MAP : Outport
  wires:
  Transfer Fcn/1 -> MAP/1
  CeR/1 -> Transfer Fcn/1

== matlab function amicas_simulator_v1/Subsystem2/Greco RSM BIS/MATLAB Function ==
  data: up input; y output; ur input; C50p input; C50r input; E0 input; Emax input; gamma input; alpha input
function y = fcn(up, ur, C50p, C50r, E0, Emax, gamma, alpha)
Ip = up/C50p;
Ir = ur/C50r;
u = Ip + Ir + alpha*Ip*Ir; 

y = E0 - (Emax) * u^gamma / (1+u^gamma);

== matlab function amicas_simulator_v1/MATLAB Function1 ==
  data: Ut input; Ur input; Ap parameter; Bp parameter; Cp parameter; Ar parameter; Br parameter; Cr parameter; Yt input; NOL input; ParamsOut output; d input; clock input
function ParamsOut = IDE_BISNOL(Ut,Ur,Ap,Bp,Cp,Ar,Br,Cr,Yt,NOL,d,clock)  
    ParamsOut = zeros(2,1);
    if ~isfinite(Ut),  Ut = 0;    end
    if ~isfinite(Ur),  Ur = 0;    end
    if ~isfinite(d),   d  = 0;    end
    Yt = Yt - d;
    if ~isfinite(Yt),  Yt = 100;  end
    if ~isfinite(NOL), NOL = 34;  end
    period_val = 10;
    Tsc = 5/60;
    if abs(10-clock) < 2*Tsc || (abs(mod(clock,period_val)) < Tsc)
        period = 1;
    else
        period = 0;
    end

    if clock > 10
        phase = 1;
    else
        phase =0;
    end

    persistent xp_k1 xr_k1 CepWindow CerWindow dWindow BISWindow NOLWindow Params ParamsOut_prev Ni
    
    if isempty(Params)
        Params = [-1; -1; 0; 1; -1; -1; 0; 1];
    
        xp_k1 = zeros(4,1);
        xr_k1 = zeros(4,1);
    
        Ni = (period_val)/Tsc;
        CepWindow = zeros(Ni,1); CerWindow = zeros(Ni,1); dWindow   = zeros(Ni,1);
        BISWindow = zeros(Ni,1); NOLWindow = zeros(Ni,1);
        ParamsOut_prev = zeros(2,1);
    end
    
    k1       = Params(1);   k2       = Params(2);   kd       = Params(3);
    bias     = Params(4);   k1_DOA   = Params(5);   k2_DOA   = Params(6);
    kd_DOA   = Params(7);   bias_DOA = Params(8);  
    
    % Default parameters (used when period == false)
    p  = [k1; k2; kd; bias];
    p2 = [k1_DOA; k2_DOA; kd_DOA; bias_DOA];
    
    xp_k = Ap*xp_k1 + Bp*Ut;    xr_k = Ar*xr_k1 + Br*Ur;
    
    xp_k(~isfinite(xp_k)) = 0;  xr_k(~isfinite(xr_k)) = 0;
    
    Cep = Cp*xp_k;  Cer = Cr*xr_k;
    
    if ~isfinite(Cep), Cep = 0; end
    if ~isfinite(Cer), Cer = 0; end
    
    xp_k1 = xp_k;   xr_k1 = xr_k;
    Cepmax = 7; Cermax = 7;
    
    Cep = Cep/Cepmax;   Cer = Cer/Cermax;
    d   = d/30; Yt  = Yt/100;
    NOL = NOL/34;
    
    CepWindow = circshift(CepWindow,-1);    CepWindow(end) = Cep;
    CerWindow = circshift(CerWindow,-1);    CerWindow(end) = Cer;
    dWindow = circshift(dWindow,-1);        dWindow(end) = d;
    BISWindow = circshift(BISWindow,-1);    BISWindow(end) = Yt;
    NOLWindow = circshift(NOLWindow,-1);    NOLWindow(end) = NOL;
    
    CepWindow(~isfinite(CepWindow)) = 0;    CerWindow(~isfinite(CerWindow)) = 0;
    dWindow(~isfinite(dWindow))     = 0;    BISWindow(~isfinite(BISWindow)) = 1;   % normalized 100
    NOLWindow(~isfinite(NOLWindow)) = 1;   % normalized 34
    
    N = Ni;
    A = [CepWindow CerWindow dWindow ones(N,1)];
    
    Y1 = BISWindow;     Y2 = NOLWindow;
    
    %% -------- BIS IDENTIFICATION --------
    H = 2 * (A' * A);  f = -2 * (A' * Y1);
    
    lb = [-2.35; -1.0; 0; 1]; % Lower bounds for [k1, k2, k3, bias]
    ub = [-0.07; -0.07; 0; 1];     % Upper bounds for [k1, k2, k3, bias]
    
    prevParams = [k1; k2; kd; bias];
    C = [eye(4); -eye(4)];   % For both upper and lower bounds
    C_custom = [1, -1, 0, 0];  % k1 - k2 < 0
    C = [C; C_custom];
    if ~phase
        deltaLimits = [prevParams + [1; 1; 0; 1]; ...
                   -(prevParams - [1; 1; 01; 1])];
        deltaLimits = [deltaLimits; 0];  % For k1 - k2 < 0
    
    else 
        deltaLimits = [prevParams + 0*[1; 0.01; 0; 0]; ...
                   -(prevParams - 1*[1; 0.01; 0; 0])];  
        deltaLimits = [deltaLimits; 0];  % For k1 - k2 < 0
    end    
    options = optimoptions('quadprog', 'Algorithm', 'active-set', 'Display', 'off');
    % Solve using quadprog
    if period
    p = quadprog(H, f, C, deltaLimits, [], [], lb, ub, prevParams, options);
    end
    
    %% -------- NOL IDENTIFICATION --------
    H = 2 * (A' * A);
    f = -2 * (A' * Y2);
    
    lb = [-2.2; -4.35; 0; 1]; % Lower bounds for [k1, k2, k3, bias]
    ub = [-0.07; -0.07; 0; 1];     % Upper bounds for [k1, k2, k3, bias]
    
    prevParams = [k1_DOA; k2_DOA; kd_DOA; bias_DOA];
    C = [eye(4); -eye(4)];   % For both upper and lower bounds
    C_custom = [-1, 1, 0, 0];  % -k1 + k2 < 0
    C = [C; C_custom];
    if ~phase
        deltaLimits = [prevParams + [1; 1; 0; 1]; ...
                   -(prevParams - [1; 1; 0; 1])];
        deltaLimits = [deltaLimits; 0];  % For k1 - k2 < 0
    
    else 
        deltaLimits = [prevParams + 0*[0.0; 1/N*0.1; 1; 0.0]; ...
                   -(prevParams - 0*[0.0; 1/N*0.1; 1; 0.0])]; 
    
        deltaLimits = [deltaLimits; 0];  % For k1 - k2 < 0
    end    
    
    % Solve using quadprog
    options = optimoptions('quadprog', 'Algorithm', 'active-set', 'Display', 'off');
    if period
    p2 = quadprog(H, f, C, deltaLimits, [], [], lb, ub, prevParams, options);
    end
    
    %% -------- SAVE PARAMETERS --------
    if period
        Params = [p; p2];
    end
 
    % always compute output from stored parameters
    k1 = Params(1); k2 = Params(2);  
    m1 = k1*100/Cepmax; m2 = k2*100/Cermax;
    
    if ~phase
        ParamsOut = [1; 1];
    else
        ParamsOut = ParamsOut_prev; 
        if period
        ParamsOut = [-m1; -m2];
        end
    end
    ParamsOut_prev = ParamsOut;
end
%
